simulink model "humbja_mostrave"  (R2016b)
settings: Solver=VariableStepAuto  StartTime=0.0  StopTime=10  MaxStep=0.01  RelTol=1e-3
libraries: simulink x2
settings Model: Creator=aidbu  LastModifiedBy=aidbu

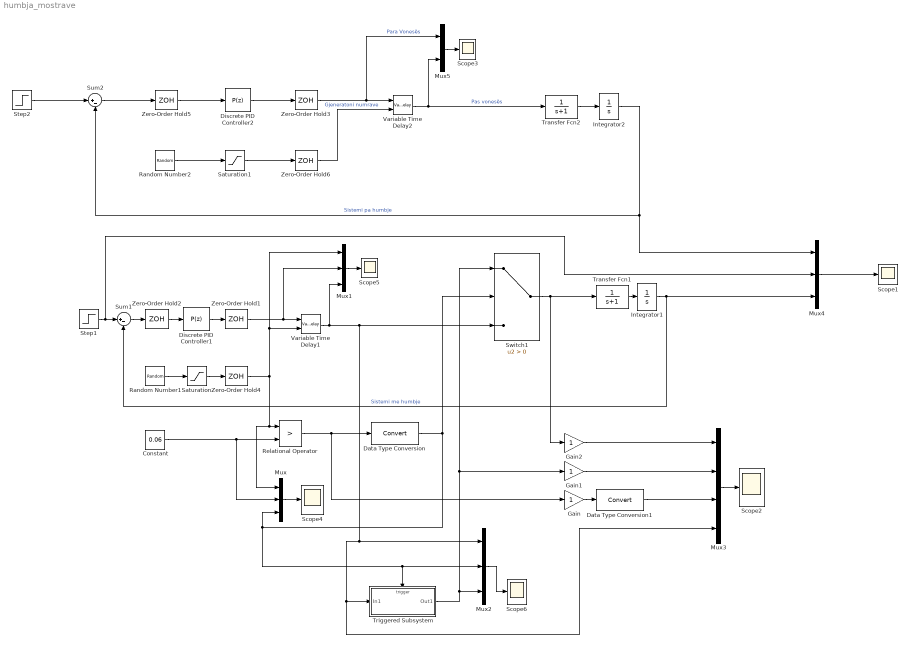
== system humbja_mostrave ==
  Constant : Constant  Value=0.06
  Data Type Conversion : DataTypeConversion
  Data Type Conversion1 : DataTypeConversion
  Discrete PID Controller1 : simulink/Continuous/PID Controller  Controller=P  TimeDomain=Discrete-time  SampleTime=0.1  IntegratorMethod=Forward Euler  FilterMethod=Forward Euler  Form=Parallel  UseFilter=on  ControllerParametersSource=internal  P=0.6159  I=0.3369  D=1.551  N=18.21  InitialConditionSource=internal  InitialConditionForIntegrator=0  InitialConditionForFilter=0  ExternalReset=none  LimitOutput=off  UpperSaturationLimit=inf  LowerSaturationLimit=-inf  LinearizeAsGain=off  AntiWindupMode=none  Kb=1  TrackingMode=off  Kt=1  PParamMin=[]  PParamMax=[]  IParamMin=[]  IParamMax=[]  DParamMin=[]  DParamMax=[]  NParamMin=[]  NParamMax=[]  KbParamMin=[]  KbParamMax=[]  KtParamMin=[]  KtParamMax=[]  POutMin=[]  POutMax=[]  IOutMin=[]  IOutMax=[]  DOutMin=[]  DOutMax=[]  NOutMin=[]  NOutMax=[]  KbOutMin=[]  KbOutMax=[]  KtOutMin=[]  KtOutMax=[]  IntegratorOutMin=[]  IntegratorOutMax=[]  FilterOutMin=[]  FilterOutMax=[]  SumOutMin=[]  SumOutMax=[]  SumI1OutMin=[]  SumI1OutMax=[]  SumI2OutMin=[]  SumI2OutMax=[]  SumI3OutMin=[]  SumI3OutMax=[]  SumDOutMin=[]  SumDOutMax=[]  SaturationOutMin=[]  SaturationOutMax=[]  IntegratorContinuousStateAttributes=''  IntegratorStateMustResolveToSignalObject=off  IntegratorRTWStateStorageClass=Auto  FilterContinuousStateAttributes=''  FilterStateMustResolveToSignalObject=off  FilterRTWStateStorageClass=Auto  DifferentiatorICPrevScaledInput=0  DifferentiatorOutMin=[]  DifferentiatorOutMax=[]
  Discrete PID Controller2 : simulink/Continuous/PID Controller  Controller=P  TimeDomain=Discrete-time  SampleTime=0.1  IntegratorMethod=Forward Euler  FilterMethod=Forward Euler  Form=Parallel  UseFilter=on  ControllerParametersSource=internal  P=0.6159  I=0.3369  D=1.551  N=18.21  InitialConditionSource=internal  InitialConditionForIntegrator=0  InitialConditionForFilter=0  ExternalReset=none  LimitOutput=off  UpperSaturationLimit=inf  LowerSaturationLimit=-inf  LinearizeAsGain=off  AntiWindupMode=none  Kb=1  TrackingMode=off  Kt=1  PParamMin=[]  PParamMax=[]  IParamMin=[]  IParamMax=[]  DParamMin=[]  DParamMax=[]  NParamMin=[]  NParamMax=[]  KbParamMin=[]  KbParamMax=[]  KtParamMin=[]  KtParamMax=[]  POutMin=[]  POutMax=[]  IOutMin=[]  IOutMax=[]  DOutMin=[]  DOutMax=[]  NOutMin=[]  NOutMax=[]  KbOutMin=[]  KbOutMax=[]  KtOutMin=[]  KtOutMax=[]  IntegratorOutMin=[]  IntegratorOutMax=[]  FilterOutMin=[]  FilterOutMax=[]  SumOutMin=[]  SumOutMax=[]  SumI1OutMin=[]  SumI1OutMax=[]  SumI2OutMin=[]  SumI2OutMax=[]  SumI3OutMin=[]  SumI3OutMax=[]  SumDOutMin=[]  SumDOutMax=[]  SaturationOutMin=[]  SaturationOutMax=[]  IntegratorContinuousStateAttributes=''  IntegratorStateMustResolveToSignalObject=off  IntegratorRTWStateStorageClass=Auto  FilterContinuousStateAttributes=''  FilterStateMustResolveToSignalObject=off  FilterRTWStateStorageClass=Auto  DifferentiatorICPrevScaledInput=0  DifferentiatorOutMin=[]  DifferentiatorOutMax=[]
  Gain : Gain
  Gain1 : Gain
  Gain2 : Gain
  Integrator1 : Integrator
  Integrator2 : Integrator
  Mux{,1..2,4} (4 alike) : Mux  Inputs=3
  Mux3 : Mux
  Mux5 : Mux  Inputs=2
  Random Number1 : RandomNumber  Mean=0.05  Variance=0.001  Seed=1  SampleTime=0.1
  Random Number2 : RandomNumber  Mean=0.05  Variance=0.001  Seed=1  SampleTime=0.1
  Relational Operator : RelationalOperator  Operator=>  OutDataTypeStr=boolean  RndMeth=Simplest
  Saturation : Saturate  UpperLimit=0.09  LowerLimit=0.01
  Saturation1 : Saturate  UpperLimit=0.09  LowerLimit=0.01
  Scope{1..6} (6 alike) : Scope
  Step1 : Step  Time=0  SampleTime=0
  Step2 : Step  Time=0  SampleTime=0
  Sum1 : Sum  Inputs=|+-
  Sum2 : Sum  Inputs=|+-
  Switch1 : Switch  Criteria=u2 > Threshold
  Transfer Fcn1 : TransferFcn  Denominator=[1 1]
  Transfer Fcn2 : TransferFcn  Denominator=[1 1]
  Triggered Subsystem : Subsystem  TreatAsAtomicUnit=on
  Variable Time Delay1 : VariableTransportDelay  MaximumDelay=0.1
  Variable Time Delay2 : VariableTransportDelay  MaximumDelay=0.1
  Zero-Order Hold{1..6} (6 alike) : ZeroOrderHold  SampleTime=0.1
  wires:
  Step1/1 -> Mux4/2, Sum1/1
  Sum1/1 -> Zero-Order Hold2/1
  Zero-Order Hold2/1 -> Discrete PID Controller1/1
  Discrete PID Controller1/1 -> Zero-Order Hold1/1
  Zero-Order Hold1/1 -> Variable Time Delay1/1, Mux1/2
  Transfer Fcn1/1 -> Integrator1/1
  Integrator1/1 -> Sum1/2, Mux4/3  "Sistemi me humbje"
  Switch1/1 -> Transfer Fcn1/1, Gain2/1
  Triggered Subsystem/1(Out1) -> Mux2/3, Gain1/1, Switch1/1
  Variable Time Delay1/1 -> Switch1/3, Mux3/4, Triggered Subsystem/1(In1), Mux2/1, Mux1/3
  Random Number1/1 -> Saturation/1
  Constant/1 -> Relational Operator/2, Mux/2
  Relational Operator/1 -> Data Type Conversion/1, Gain/1
  Gain/1 -> Data Type Conversion1/1
  Gain1/1 -> Mux3/2
  Mux/1 -> Scope4/1
  Data Type Conversion/1 -> Mux/3, Triggered Subsystem/Trigger, Mux2/2, Switch1/2
  Mux1/1 -> Scope5/1
  Zero-Order Hold4/1 -> Mux/1, Relational Operator/1, Mux1/1, Variable Time Delay1/2
  Saturation/1 -> Zero-Order Hold4/1
  Mux2/1 -> Scope6/1
  Gain2/1 -> Mux3/1
  Mux3/1 -> Scope2/1
  Data Type Conversion1/1 -> Mux3/3
  Mux4/1 -> Scope1/1
  Step2/1 -> Sum2/1
  Sum2/1 -> Zero-Order Hold5/1
  Zero-Order Hold5/1 -> Discrete PID Controller2/1
  Discrete PID Controller2/1 -> Zero-Order Hold3/1
  Zero-Order Hold3/1 -> Mux5/1, Variable Time Delay2/1  "Para Vonesës"
  Transfer Fcn2/1 -> Integrator2/1
  Integrator2/1 -> Mux4/1, Sum2/2  "Sistemi pa humbje"
  Variable Time Delay2/1 -> Mux5/2, Transfer Fcn2/1  "Pas vonesës"
  Random Number2/1 -> Saturation1/1
  Mux5/1 -> Scope3/1
  Zero-Order Hold6/1 -> Variable Time Delay2/2  "Gjeneratoni numrave"
  Saturation1/1 -> Zero-Order Hold6/1

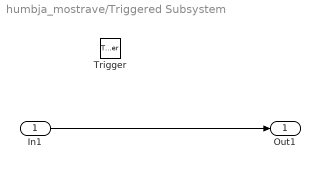
== system humbja_mostrave/Triggered Subsystem ==
  In1 : Inport
  Trigger : TriggerPort  VariantControl=Variant
  Out1 : Outport
  wires:
  In1/1 -> Out1/1
